simulink model "Q1_t"  (R2021b)
settings: Solver=VariableStepAuto  StartTime=0.0  StopTime=20  RelTol=1e-3
settings Model: Creator=nima8  LastModifiedBy=nima8

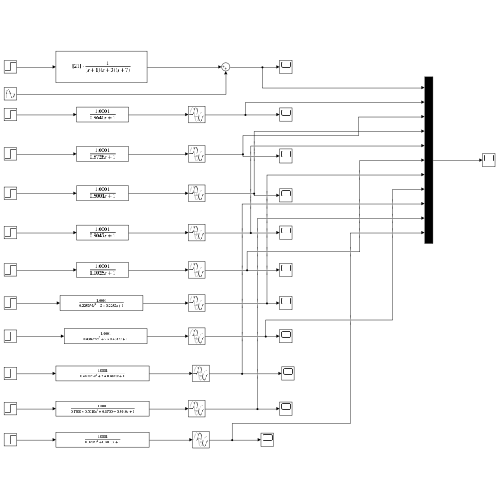
[thumbnail: Simulink's stored preview of the top-level diagram]
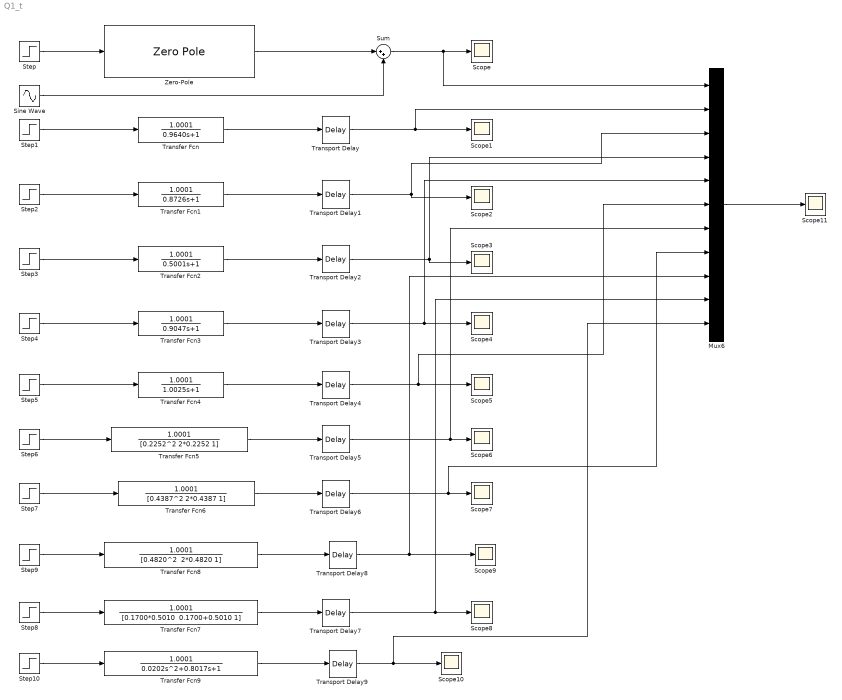
== system Q1_t ==
  Mux6 : Mux  Inputs=11
  Scope{,1..11} (12 alike) : Scope
  Sine Wave : Sin  Amplitude=0.05  Frequency=40  SampleTime=0
  Step{,1..10} (11 alike) : Step  Time=0  SampleTime=0
  Sum : Sum  Inputs=|++
  Transfer Fcn : TransferFcn  Numerator=[1.0001]  Denominator=[0.9640 1]
  Transfer Fcn1 : TransferFcn  Numerator=[1.0001]  Denominator=[0.8726 1]
  Transfer Fcn2 : TransferFcn  Numerator=[1.0001]  Denominator=[0.5001 1]
  Transfer Fcn3 : TransferFcn  Numerator=[1.0001]  Denominator=[0.9047 1]
  Transfer Fcn4 : TransferFcn  Numerator=[1.0001]  Denominator=[1.0025 1]
  Transfer Fcn5 : TransferFcn  Numerator=[1.0001]  Denominator=[0.2252^2 2*0.2252 1]
  Transfer Fcn6 : TransferFcn  Numerator=[1.0001]  Denominator=[0.4387^2 2*0.4387 1]
  Transfer Fcn7 : TransferFcn  Numerator=[1.0001]  Denominator="[0.1700*0.5010  0.1700+0.5010 1]"
  Transfer Fcn8 : TransferFcn  Numerator=[1.0001]  Denominator="[0.4820^2  2*0.4820 1]"
  Transfer Fcn9 : TransferFcn  Numerator=[1.0001]  Denominator="[0.0202  0.8017 1]"
  Transport Delay{,1..6,8} (8 alike) : TransportDelay  DelayTime=0.5120
  Transport Delay7 : TransportDelay  DelayTime=0.4262
  Transport Delay9 : TransportDelay  DelayTime=0.6744
  Zero-Pole : ZeroPole  Zeros=[]  Poles="[-1  -3  -7]"  Gain=[21]
  wires:
  Step/1 -> Zero-Pole/1
  Zero-Pole/1 -> Sum/1
  Sum/1 -> Mux6/1, Scope/1
  Sine Wave/1 -> Sum/2
  Transfer Fcn/1 -> Transport Delay/1
  Transport Delay/1 -> Mux6/2, Scope1/1
  Transfer Fcn1/1 -> Transport Delay1/1
  Transfer Fcn2/1 -> Transport Delay2/1
  Step4/1 -> Transfer Fcn3/1
  Transfer Fcn4/1 -> Transport Delay4/1
  Transport Delay2/1 -> Scope3/1, Mux6/4
  Step1/1 -> Transfer Fcn/1
  Step2/1 -> Transfer Fcn1/1
  Step3/1 -> Transfer Fcn2/1
  Transport Delay3/1 -> Scope4/1, Mux6/5
  Transport Delay4/1 -> Scope5/1, Mux6/6
  Step5/1 -> Transfer Fcn4/1
  Transfer Fcn3/1 -> Transport Delay3/1
  Mux6/1 -> Scope11/1
  Transport Delay1/1 -> Mux6/3, Scope2/1
  Transfer Fcn5/1 -> Transport Delay5/1
  Step6/1 -> Transfer Fcn5/1
  Transport Delay5/1 -> Mux6/7, Scope6/1
  Transfer Fcn6/1 -> Transport Delay6/1
  Transport Delay6/1 -> Mux6/8, Scope7/1
  Step7/1 -> Transfer Fcn6/1
  Step8/1 -> Transfer Fcn7/1
  Transfer Fcn7/1 -> Transport Delay7/1
  Transport Delay7/1 -> Mux6/10, Scope8/1
  Step9/1 -> Transfer Fcn8/1
  Transfer Fcn8/1 -> Transport Delay8/1
  Transport Delay8/1 -> Mux6/9, Scope9/1
  Step10/1 -> Transfer Fcn9/1
  Transfer Fcn9/1 -> Transport Delay9/1
  Transport Delay9/1 -> Mux6/11, Scope10/1
